simulink model "q3"  (R2019a)
settings: Solver=VariableStepAuto  StartTime=0.0  StopTime=0.5  RelTol=1e-3
settings Model: Creator=ADMIN  LastModifiedBy=ADMIN

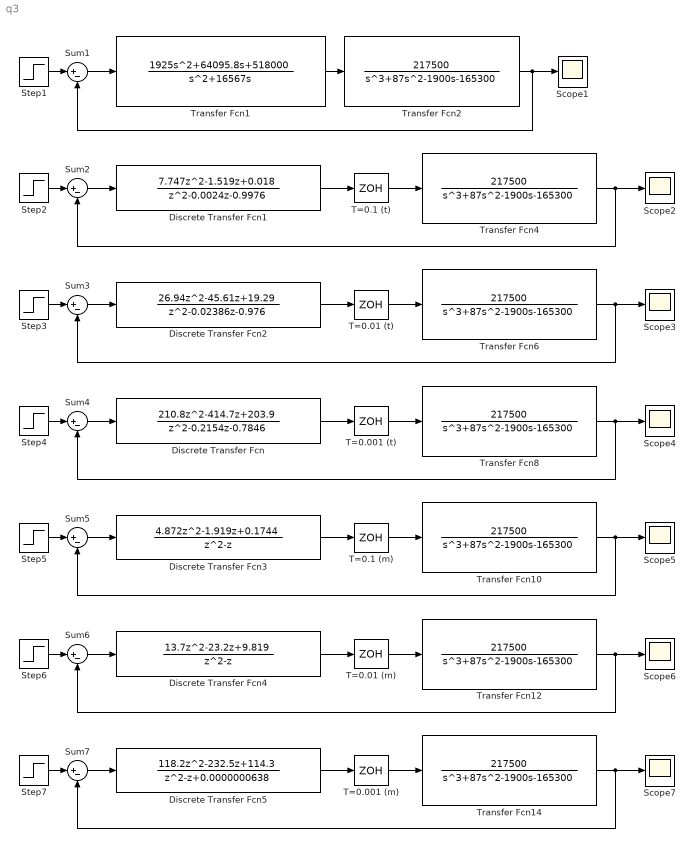
== system q3 ==
  Discrete Transfer Fcn : DiscreteTransferFcn  Numerator=[210.8 -414.7 203.9]  Denominator=[1 -0.2154 -0.7846]  SampleTime=0.001
  Discrete Transfer Fcn1 : DiscreteTransferFcn  Numerator=[7.747 -1.519 0.018]  Denominator=[1 -0.0024 -0.9976]  SampleTime=0.1
  Discrete Transfer Fcn2 : DiscreteTransferFcn  Numerator=[26.94 -45.61 19.29]  Denominator=[1 -0.02386 -0.976]  SampleTime=0.01
  Discrete Transfer Fcn3 : DiscreteTransferFcn  Numerator=[4.872 -1.919 0.1744]  Denominator=[1 -1 0]  SampleTime=0.1
  Discrete Transfer Fcn4 : DiscreteTransferFcn  Numerator=[13.7 -23.2 9.819]  Denominator=[1 -1 0]  SampleTime=0.01
  Discrete Transfer Fcn5 : DiscreteTransferFcn  Numerator=[118.2 -232.5 114.3]  Denominator=[1 -1 0.0000000638]  SampleTime=0.001
  Scope{1..7} (7 alike) : Scope
  Step1 : Step  Time=0  SampleTime=0
  Step2 : Step  Time=0  SampleTime=0.1
  Step3 : Step  Time=0  SampleTime=0.01
  Step4 : Step  Time=0  SampleTime=0.001
  Step5 : Step  Time=0  SampleTime=0.1
  Step6 : Step  Time=0  SampleTime=0.01
  Step7 : Step  Time=0  SampleTime=0.001
  Sum{1..7} (7 alike) : Sum  Inputs=|+-
  T=0.001 (m) : ZeroOrderHold  SampleTime=0.001
  T=0.001 (t) : ZeroOrderHold  SampleTime=0.001
  T=0.01 (m) : ZeroOrderHold  SampleTime=0.01
  T=0.01 (t) : ZeroOrderHold  SampleTime=0.01
  T=0.1 (m) : ZeroOrderHold  SampleTime=0.1
  T=0.1 (t) : ZeroOrderHold  SampleTime=0.1
  Transfer Fcn1 : TransferFcn  Numerator=[1925 64095.8 518000]  Denominator=[1 16567 0]
  Transfer Fcn{2,4,6,8,10,12,14} (7 alike) : TransferFcn  Numerator=[217500]  Denominator=[1 87 -1900 -165300]
  wires:
  Transfer Fcn1/1 -> Transfer Fcn2/1
  Step1/1 -> Sum1/1
  Transfer Fcn2/1 -> Sum1/2, Scope1/1
  Sum1/1 -> Transfer Fcn1/1
  Sum2/1 -> Discrete Transfer Fcn1/1
  Transfer Fcn4/1 -> Sum2/2, Scope2/1
  Step2/1 -> Sum2/1
  Discrete Transfer Fcn1/1 -> T=0.1 (t)/1
  T=0.1 (t)/1 -> Transfer Fcn4/1
  Sum3/1 -> Discrete Transfer Fcn2/1
  T=0.01 (t)/1 -> Transfer Fcn6/1
  Step3/1 -> Sum3/1
  Discrete Transfer Fcn2/1 -> T=0.01 (t)/1
  Transfer Fcn6/1 -> Sum3/2, Scope3/1
  Sum4/1 -> Discrete Transfer Fcn/1
  T=0.001 (t)/1 -> Transfer Fcn8/1
  Step4/1 -> Sum4/1
  Discrete Transfer Fcn/1 -> T=0.001 (t)/1
  Transfer Fcn8/1 -> Sum4/2, Scope4/1
  Transfer Fcn10/1 -> Sum5/2, Scope5/1
  Sum5/1 -> Discrete Transfer Fcn3/1
  T=0.1 (m)/1 -> Transfer Fcn10/1
  Sum7/1 -> Discrete Transfer Fcn5/1
  Step6/1 -> Sum6/1
  Discrete Transfer Fcn4/1 -> T=0.01 (m)/1
  Transfer Fcn12/1 -> Sum6/2, Scope6/1
  Discrete Transfer Fcn3/1 -> T=0.1 (m)/1
  Transfer Fcn14/1 -> Sum7/2, Scope7/1
  Sum6/1 -> Discrete Transfer Fcn4/1
  Discrete Transfer Fcn5/1 -> T=0.001 (m)/1
  T=0.01 (m)/1 -> Transfer Fcn12/1
  Step7/1 -> Sum7/1
  Step5/1 -> Sum5/1
  T=0.001 (m)/1 -> Transfer Fcn14/1
